simulink model "Lab2tepo"  (R2017b)
settings: Solver=VariableStepAuto  StartTime=0.0  StopTime=50  RelTol=1e-3
values from neighbouring files (symbols this model uses):
  Fg1 = m1*g*sin(alpha)    [lab2_data.m]
  Fg2 = m2*g*sin(alpha)    [lab2_data.m]
  kdmp = 1.5    [Labdata.m]    (also in lab2_data.m = 2)
  ksp = 12    [Labdata.m]    (also in lab2_data.m = 20)
  m1 = 200    [lab2_data.m]
  m2 = 50    [lab2_data.m]
undefined symbols (not defined in the file or in its folder): F
libraries: fl_lib x11, nesl_utility x8
settings Model: Creator=Aleksandr  LastModifiedBy=Aleksandr

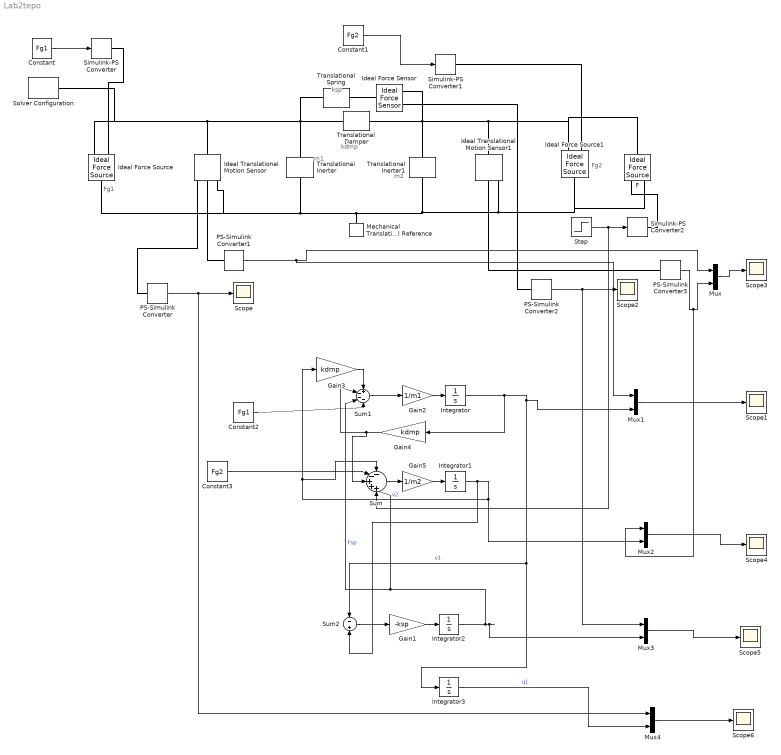
== system Lab2tepo ==
  note: Fg2
  note: Fg1
  note: m2
  note: m1
  note: kdmp
  note: ksp
  Constant : Constant  Value=Fg1
  Constant1 : Constant  Value=Fg2
  Constant2 : Constant  Value=Fg1
  Constant3 : Constant  Value=Fg2
  F : fl_lib/Mechanical/Mechanical Sources/Ideal Force Source
  Gain1 : Gain  Gain=-ksp
  Gain2 : Gain  Gain=1/m1
  Gain3 : Gain  Gain=kdmp
  Gain4 : Gain  Gain=kdmp
  Gain5 : Gain  Gain=1/m2
  Ideal Force Sensor : fl_lib/Mechanical/Mechanical Sensors/Ideal Force Sensor
  Ideal Force Source : fl_lib/Mechanical/Mechanical Sources/Ideal Force Source
  Ideal Force Source1 : fl_lib/Mechanical/Mechanical Sources/Ideal Force Source
  Ideal Translational Motion Sensor : fl_lib/Mechanical/Mechanical Sensors/Ideal Translational Motion Sensor  offset=0 m
  Ideal Translational Motion Sensor1 : fl_lib/Mechanical/Mechanical Sensors/Ideal Translational Motion Sensor  offset=0 m
  Integrator : Integrator
  Integrator1 : Integrator
  Integrator2 : Integrator  InitialCondition=0.1*ksp
  Integrator3 : Integrator
  Mechanical Translational Reference : fl_lib/Mechanical/Translational Elements/Mechanical Translational Reference
  Mux{,1..4} (5 alike) : Mux  Inputs=2
  PS-Simulink Converter{,1..3} (4 alike) : nesl_utility/PS-Simulink Converter  PhysicalDomain=network_engine_domain  SubClassName=ps_output  LeftPortType=input  RightPortType=output  PseudoPeriodic=off  Frequencies=[]  Unit=1  AffineConversion=off
  Scope{,1..6} (7 alike) : Scope
  Simulink-PS Converter : nesl_utility/Simulink-PS Converter  PhysicalDomain=network_engine_domain  SubClassName=ps_input  LeftPortType=input  RightPortType=output  PseudoPeriodic=off  Frequencies=[]  NoiseDistribution=none  NoiseParameters=[]  Unit=1  AffineConversion=off  FilteringAndDerivatives=provide  SimscapeFilterOrder=1  InputFilterTimeConstant=0.001  UdotUserProvided=0
  Simulink-PS Converter1 : nesl_utility/Simulink-PS Converter  PhysicalDomain=network_engine_domain  SubClassName=ps_input  LeftPortType=input  RightPortType=output  PseudoPeriodic=off  Frequencies=[]  NoiseDistribution=none  NoiseParameters=[]  Unit=1  AffineConversion=off  FilteringAndDerivatives=provide  SimscapeFilterOrder=1  InputFilterTimeConstant=0.001  UdotUserProvided=0
  Simulink-PS Converter2 : nesl_utility/Simulink-PS Converter  PhysicalDomain=network_engine_domain  SubClassName=ps_input  LeftPortType=input  RightPortType=output  PseudoPeriodic=off  Frequencies=[]  NoiseDistribution=none  NoiseParameters=[]  Unit=1  AffineConversion=off  FilteringAndDerivatives=provide  SimscapeFilterOrder=1  InputFilterTimeConstant=0.001  UdotUserProvided=0
  Solver Configuration : nesl_utility/Solver Configuration  PhysicalDomain=network_engine_domain  SubClassName=solver  LeftPortType=input  RightPortType=generic  Accelerate=off  Tones=[]  Harmonics=[]  SimulateNoise=off  Profile=off  UseLocalSampling=off  EnableSwitchedLinearOptims=on  FrequencyDomain=off  UseCCode=off  RelTol=0.001  AbsTol=1e-06  MinStep=1e-09  ToWorkspace=off  RevertToSquareIcSolve=off  NumHomotopyIterations=100  PhasorMode=off  PhasorModeNumHarmonics=1  DoDC=off  ResidualTolerance=1e-09  UseLocalSolver=off  LocalSolverChoice=NE_BACKWARD_EULER_ADVANCER  LocalSolverSampleTime=0.001  DoFixedCost=off  MaxNonlinIter=3  MaxModeIter=2  LinearAlgebra=Sparse  DelaysMemoryBudget=1024  AutomaticFiltering=on  FilteringTimeConstant=0.001
  Step : Step  After=F  SampleTime=0
  Sum : Sum  Inputs=--+++
  Sum1 : Sum  Inputs=+---
  Sum2 : Sum  Inputs=-+
  Translational Inerter : fl_lib/Mechanical/Translational Elements/Translational Inerter  B=m1 kg  v_specify=off  v_priority=High  v=0 m/s  v_nominal_specify=off  v_nominal_unit=m/s  v_nominal_value=1  f_specify=off  f_priority=None  f=0 N  f_nominal_specify=off  f_nominal_unit=N  f_nominal_value=1
      settings: SourceProductName=Simscape  SourceProductBaseCode=SS
  Translational Inerter1 : fl_lib/Mechanical/Translational Elements/Translational Inerter  B=m2 kg  v_specify=off  v_priority=High  v=0 m/s  v_nominal_specify=off  v_nominal_unit=m/s  v_nominal_value=1  f_specify=off  f_priority=None  f=0 N  f_nominal_specify=off  f_nominal_unit=N  f_nominal_value=1
      settings: SourceProductName=Simscape  SourceProductBaseCode=SS
  Translational Damper : fl_lib/Mechanical/Translational Elements/Translational Damper  D=kdmp N/(m/s)  v_specify=off  v_priority=None  v=0 m/s  v_nominal_specify=off  v_nominal_unit=m/s  v_nominal_value=1  f_specify=off  f_priority=None  f=0 N  f_nominal_specify=off  f_nominal_unit=N  f_nominal_value=1
  Translational Spring : fl_lib/Mechanical/Translational Elements/Translational Spring  spr_rate=ksp N/m  v_specify=off  v_priority=None  v=0 m/s  v_nominal_specify=off  v_nominal_unit=m/s  v_nominal_value=1  f_specify=off  f_priority=None  f=0 N  f_nominal_specify=off  f_nominal_unit=N  f_nominal_value=1  x_specify=on  x_priority=High  x=0.1 m  x_nominal_specify=off  x_nominal_unit=m  x_nominal_value=1
  wires:
  Constant/1 -> Simulink-PS Converter/1
  Constant1/1 -> Simulink-PS Converter1/1
  PS-Simulink Converter/1 -> Mux4/1, Scope/1
  PS-Simulink Converter1/1 -> Mux1/1, Mux/1
  PS-Simulink Converter2/1 -> Mux3/1, Scope2/1
  PS-Simulink Converter3/1 -> Mux2/1, Mux/2
  Mux/1 -> Scope3/1
  Sum1/1 -> Gain2/1
  Sum/1 -> Gain5/1
  Sum2/1 -> Gain1/1
  Integrator/1 -> Gain4/1, Mux1/2, Sum2/1, Integrator3/1  "v1"
  Integrator1/1 -> Sum2/2, Mux2/2, Sum/1, Gain3/1  "v2"
  Integrator2/1 -> Sum/4, Sum1/3, Mux3/2  "Fsp"
  Integrator3/1 -> Mux4/2  "q1"
  Gain1/1 -> Integrator2/1
  Gain2/1 -> Integrator/1
  Gain3/1 -> Sum1/1
  Gain4/1 -> Sum/3, Sum1/2
  Constant2/1 -> Sum1/4
  Constant3/1 -> Sum/2
  Step/1 -> Sum/5, Simulink-PS Converter2/1
  Gain5/1 -> Integrator1/1
  Mux1/1 -> Scope1/1
  Mux2/1 -> Scope4/1
  Mux3/1 -> Scope5/1
  Mux4/1 -> Scope6/1
  connections:
  Mechanical Translational Reference/LConn1 -- Ideal Translational Motion Sensor1/RConn1 -- F/RConn2 -- Ideal Force Source1/LConn1 -- Translational Inerter1/RConn1 -- Ideal Translational Motion Sensor/RConn1 -- Ideal Force Source/LConn1 -- Translational Inerter/RConn1
  Translational Inerter/LConn1 -- Ideal Translational Motion Sensor/LConn1 -- Solver Configuration/RConn1 -- Ideal Force Source/RConn2 -- Translational Damper/LConn1 -- Translational Spring/LConn1
  Translational Inerter1/LConn1 -- Ideal Force Sensor/RConn1 -- Ideal Translational Motion Sensor1/LConn1 -- F/LConn1 -- Ideal Force Source1/RConn2 -- Translational Damper/RConn1
  Simulink-PS Converter/RConn1 -- Ideal Force Source/RConn1
  Simulink-PS Converter1/RConn1 -- Ideal Force Source1/RConn1
  F/RConn1 -- Simulink-PS Converter2/RConn1
  Ideal Force Sensor/LConn1 -- Translational Spring/RConn1
  PS-Simulink Converter/LConn1 -- Ideal Translational Motion Sensor/RConn3
  PS-Simulink Converter1/LConn1 -- Ideal Translational Motion Sensor/RConn2
  PS-Simulink Converter2/LConn1 -- Ideal Force Sensor/RConn2
  PS-Simulink Converter3/LConn1 -- Ideal Translational Motion Sensor1/RConn2
